simulink model "HbridgeWithDeadTime"  (R2019b)
settings: Solver=VariableStepAuto  StartTime=0.0  StopTime=0.1  RelTol=1e-3
libraries: powerlib x12, powerlib_meascontrol x1
settings Model: Creator=FAST  LastModifiedBy=FAST

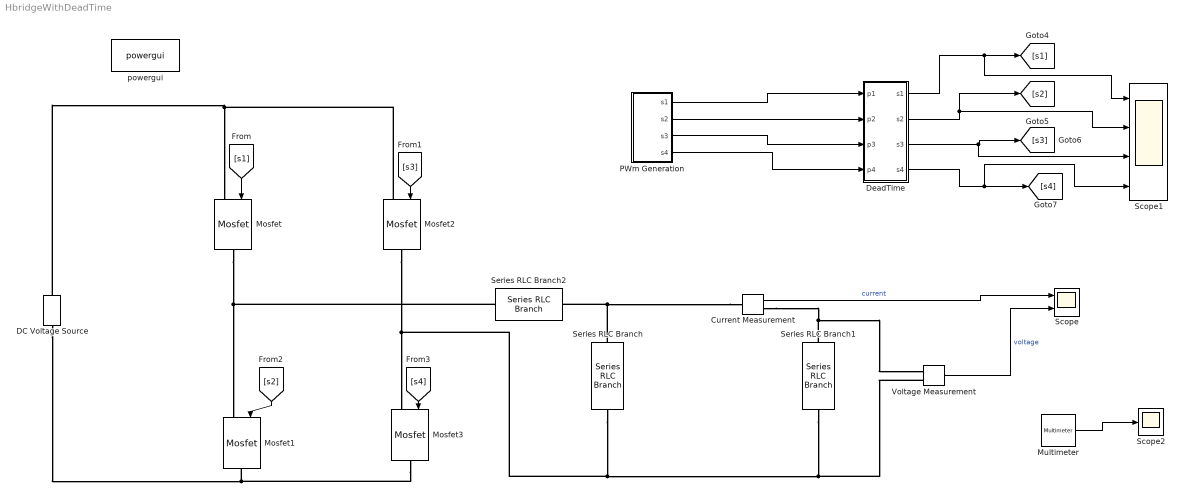
== system HbridgeWithDeadTime ==
  Current Measurement : powerlib/Measurements/Current Measurement  PhasorSimulation=off  OutputType=Complex  PSBequivalent=0
      settings: SourceProductName=Simscape Electrical
  DC Voltage Source : powerlib/Electrical Sources/DC Voltage Source  Amplitude=60  Measurements=None
      settings: SourceProductName=Simscape Electrical
  DeadTime : Subsystem  mask(DeadTime){freq=50, deadTime=45e-6}
      mask prompts: freq "Frequency (Hz)"
      mask help:
      | This block adds dead time to the input  for pwm inverters.
      | implemented with stateflow chart.
      | it adds given deadtime after every half period minus deadtime.
  Mosfet{,1..3} (4 alike) : powerlib/Power Electronics/Mosfet  Ron=0.1  Lon=0  Rd=0.01  Vfd=0  IC=0  Rs=1e5  Cs=inf  Measurements=off
      settings: SourceProductName=Simscape Electrical
  Multimeter : powerlib/Measurements/Multimeter  PhasorSimulation=off  OutputType=Complex  sel=1  L=1  Gain=1  yselected={'Ib: Series RLC Branch1'};  PSBOutputType=1  PSBequivalent=0  AxesSetting=[0,0.1,-100,100]  Display=0  SavedBlockNames=-11
      settings: SourceProductName=Simscape Electrical
  PWm Generation : Subsystem
  Scope : Scope  NumInputPorts=2
  Scope1 : Scope  NumInputPorts=4
  Scope2 : Scope
  Series RLC Branch : powerlib/Elements/Series RLC Branch  LConnTagsString=__new0  RConnTagsString=__new0  BranchType=C  Resistance=0.0042  Inductance=1e-3  SetiL0=off  InitialCurrent=0  Capacitance=2e-6  Setx0=off  InitialVoltage=0  Measurements=None
      settings: SourceProductName=Simscape Electrical
  Series RLC Branch1 : powerlib/Elements/Series RLC Branch  LConnTagsString=__new0  RConnTagsString=__new0  BranchType=R  Resistance=15  Inductance=1e-3  SetiL0=off  InitialCurrent=0  Capacitance=4.4e-6  Setx0=off  InitialVoltage=0  Measurements=Branch current
      settings: SourceProductName=Simscape Electrical
  Series RLC Branch2 : powerlib/Elements/Series RLC Branch  LConnTagsString=__new0  RConnTagsString=__new0  BranchType=L  Resistance=0.001  Inductance=3.6e-3  SetiL0=off  InitialCurrent=0  Capacitance=2200e-6  Setx0=off  InitialVoltage=0  Measurements=None
      settings: SourceProductName=Simscape Electrical
  Voltage Measurement : powerlib/Measurements/Voltage Measurement  PhasorSimulation=off  OutputType=Complex  PSBequivalent=0
      settings: SourceProductName=Simscape Electrical
  powergui : powerlib/powergui  Priority=1  SimulationMode=Continuous  SampleTime=50e-6  frequency=60  Iterations=50  frequencyindice=0  Pbase=100e6  ErrMax=1e-4  UnitsV=kV  UnitsW=MW  buscounter=0  FunctionMessages=off  echomessages=off  EnableUseOfTLC=off  CurrentSourceSwitches=off  DisableSnubberDevices=off  DisableRonSwitches=off  DisableVfSwitches=off  DisplayEquations=off  AutomaticDiscreteSolvers=off  SolverType=Tustin/Backward Euler (TBE)  Interpol=off  ExternalGateDelay=off  methode=off  Ts=100  x0status=blocks  SPID=on  SwTol=0  HookPort=off  NonlinearTolerance=1e-4  nMaxIteration=100  ContinueOnMaxIteration=off  RestoreLinks=warning  ResistiveCurrentMeasurement=off  Frange=[0:2:500]  Ylog=off  Xlog=on  ShowGrid=off  save=off  variable=ZData  structure=current  ZoomFFT=off  StartTime=0.01  cycles=4  DisplayStyle=1  fundamental=50  FreqAxis=off  MaxFrequency=300  frequencyindicesteady=1  RmsSteady=1  display=off
      settings: SourceProductName=Simscape Electrical
  wires:
  [s3] -> Mosfet2/1
  [s4] -> Mosfet3/1
  [s1] -> Mosfet/1
  [s2] -> Mosfet1/1
  Current Measurement/1 -> Scope/1  "current"
  Voltage Measurement/1 -> Scope/2  "voltage"
  PWm Generation/1(s1) -> DeadTime/1(p1)
  PWm Generation/2(s2) -> DeadTime/2(p2)
  PWm Generation/3(s3) -> DeadTime/3(p3)
  PWm Generation/4(s4) -> DeadTime/4(p4)
  DeadTime/1(s1) -> Scope1/1, [s1]
  DeadTime/2(s2) -> Scope1/2, [s2]
  DeadTime/3(s3) -> Scope1/3, [s3]
  DeadTime/4(s4) -> Scope1/4, [s4]
  Multimeter/1 -> Scope2/1
  connections:
  DC Voltage Source/RConn1 -- Mosfet2/LConn1 -- Mosfet/LConn1
  DC Voltage Source/LConn1 -- Mosfet3/RConn1 -- Mosfet1/RConn1
  Mosfet2/RConn1 -- Series RLC Branch/RConn1 -- Series RLC Branch1/RConn1 -- Voltage Measurement/LConn2 -- Mosfet3/LConn1
  Series RLC Branch1/LConn1 -- Current Measurement/RConn1 -- Voltage Measurement/LConn1
  Series RLC Branch2/RConn1 -- Mosfet1/LConn1 -- Mosfet/RConn1
  Series RLC Branch/LConn1 -- Current Measurement/LConn1 -- Series RLC Branch2/LConn1

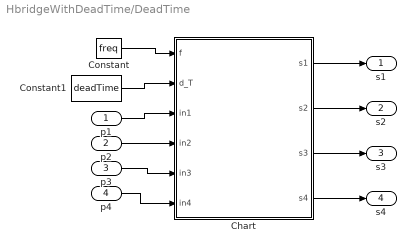
== system HbridgeWithDeadTime/DeadTime ==
  p1 : Inport
  p2 : Inport  Port=2
  p3 : Inport  Port=3
  p4 : Inport  Port=4
  Chart : Stateflow chart  BlockKeywords=__PRM__SERIALIZED__DATA__:Stateflow Chart,Stateflow Diagram  TreatAsAtomicUnit=on
  Constant : Constant  Value=freq
  Constant1 : Constant  Value=deadTime  OutDataTypeStr=double
  s1 : Outport
  s2 : Outport  Port=2
  s3 : Outport  Port=3
  s4 : Outport  Port=4
  wires:
  Chart/1(s1) -> s1/1
  p2/1 -> Chart/4(in2)
  Chart/2(s2) -> s2/1
  p3/1 -> Chart/5(in3)
  Constant/1 -> Chart/1(f)
  Chart/4(s4) -> s4/1
  Constant1/1 -> Chart/2(d_T)
  Chart/3(s3) -> s3/1
  p1/1 -> Chart/3(in1)
  p4/1 -> Chart/6(in4)

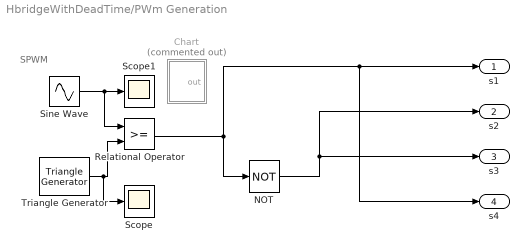
== system HbridgeWithDeadTime/PWm Generation ==
  note: SPWM
  Chart : Stateflow chart  Commented=on  BlockKeywords=__PRM__SERIALIZED__DATA__:Stateflow Chart,Stateflow Diagram  TreatAsAtomicUnit=on
  NOT : Logic  Operator=NOT  IconShape=distinctive  AllPortsSameDT=off  OutDataTypeStr=boolean
  Relational Operator : RelationalOperator  OutDataTypeStr=boolean  RndMeth=Simplest
  Scope : Scope
  Scope1 : Scope
  Sine Wave : Sin  Frequency=2*pi*50  SampleTime=0
  Triangle Generator : powerlib_meascontrol/Pulse & Signal Generators/Triangle Generator  Freq=20e3  Phase=90  Ts=0
      settings: SourceProductName=Simscape Electrical
  s1 : Outport
  s2 : Outport  Port=2
  s3 : Outport  Port=3
  s4 : Outport  Port=4
  wires:
  Triangle Generator/1 -> Scope/1, Relational Operator/2
  Sine Wave/1 -> Scope1/1, Relational Operator/1
  NOT/1 -> s3/1, s2/1
  Relational Operator/1 -> s4/1, s1/1, NOT/1

== stateflow chart HbridgeWithDeadTime/PWm Generation/Chart ==
  state on
    out=true;
  state off
    out=false;
  (default) -> on
  on -> off : after(10e-3,sec)
  off -> on : after(10e-3,sec)
  data: out output

== stateflow chart HbridgeWithDeadTime/DeadTime/Chart ==
  state main
    T1=(1/f)/2-d_T;
    s1=in1;
    s2=in2
    s3=in3;
    s4=in4;
  state DeadTime
    s1=false;
    s2=false;
    s3=false;
    s4=false;
  (default) -> main
  main -> DeadTime : after(T1,sec)
  DeadTime -> main : after(d_T,sec)
  data: f input double; d_T input double; in1 input boolean; in2 input boolean; in3 input boolean; in4 input boolean; s1 output boolean; s2 output boolean; s3 output boolean; s4 output boolean; T1 local double
